simulink model "project_1"  (R2015b)
settings: Solver=ode15s  StartTime=0  StopTime=2000  FixedStep=1e-3  RelTol=1e-4
undefined symbols (not defined in the file): Kd_surge, Kd_sway, Kd_yaw, Ki_surge, Ki_sway, Ki_yaw, Kp_surge, Kp_sway, Kp_yaw, Par, Sim
libraries: marine_gnc x2
settings Model: Creator=torstebo  LastModifiedBy=ShivJeet
settings SolverCC: MaxConsecutiveMinStep=3  SolverJacobianMethodControl=FullPerturbation  ZeroCrossControl=DisableAll  ZeroCrossAlgorithm=Adaptive
settings DataIOCC: Decimation=10  InitialState=xFinal  LimitDataPoints=off  SaveFormat=StructureWithTime  SaveOutput=off  InspectSignalLogs=on  VisualizeSimOutput=off  SaveTime=off
settings OptimizationCC: AccelVerboseBuild=on
settings DebuggingCC: AlgebraicLoopMsg=error  UnderspecifiedInitializationDetection=Classic  MergeDetectMultiDrivingBlocksExec=none  SolverPrmCheckMsg=warning  StateNameClashWarn=warning
settings HardwareCC: ProdBitPerPointer=32  ProdLargestAtomicFloat=None  ProdIntDivRoundTo=Undefined  ProdEndianess=Unspecified  ProdWordSize=32  ProdHWDeviceType=32-bit Generic
settings GRTTargetCC: GeneratePreprocessorConditionals=Disable all
settings ConfigComp: CovModelRefEnable=Off  CovSFcnEnable=off

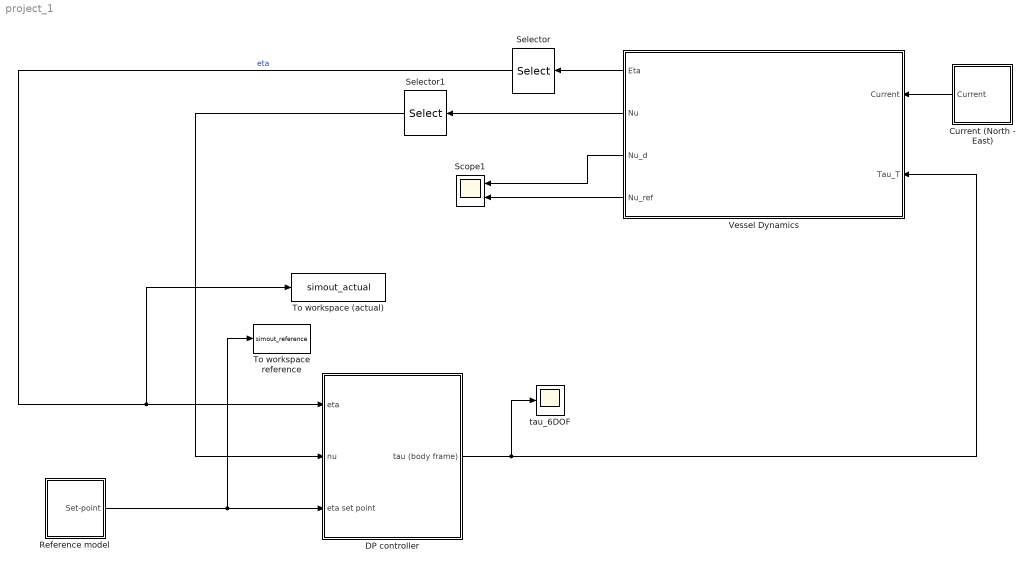
== system project_1 ==
  Current (North - East) : Subsystem
  DP controller : Subsystem
  Reference model : Subsystem
  Scope1 : Scope  NumInputPorts=2
  Selector : Selector  InputPortWidth=6  IndexOptions=Index vector (dialog)  Indices=[1 2 6]  OutputSizes=1
  Selector1 : Selector  InputPortWidth=6  IndexOptions=Index vector (dialog)  Indices=[1 2 6]  OutputSizes=1
  To workspace (actual) : ToWorkspace  VariableName=simout_actual  SaveFormat=Timeseries  SampleTime=-1
  To workspace reference : ToWorkspace  VariableName=simout_reference  SaveFormat=Timeseries  SampleTime=-1
  Vessel Dynamics : Subsystem
      mask Display:
      | image(imread('Files/supply.jpg'))
      | color('black'); port_label('output', 1, 'eta')
      | color('black'); port_label('output', 2, 'nu')
      | color('black'); port_label('output', 3, 'nu_d')
      | color('black'); port_label('output', 4, 'nu_ref')
      | color('black'); port_label('input', 1, 'nu_c')
      | color('black'); port_label('input', 2, 'tau')
  tau_6DOF : Scope
  wires:
  Vessel Dynamics/1(Eta) -> Selector/1
  Vessel Dynamics/2(Nu) -> Selector1/1
  Current (North - East)/1(Current) -> Vessel Dynamics/1(Current)
  DP controller/1(tau (body frame)) -> tau_6DOF/1, Vessel Dynamics/2(Tau_T)
  Reference model/1(Set-point) -> To workspace reference/1, DP controller/3(eta set point)
  Selector1/1 -> DP controller/2(nu)
  Vessel Dynamics/3(Nu_d) -> Scope1/1
  Vessel Dynamics/4(Nu_ref) -> Scope1/2
  Selector/1 -> To workspace (actual)/1, DP controller/1(eta)  "eta"

== system project_1/Current (North - East) ==
  Constant : Constant  Value=[0 0]
  Current : Outport
  wires:
  Constant/1 -> Current/1

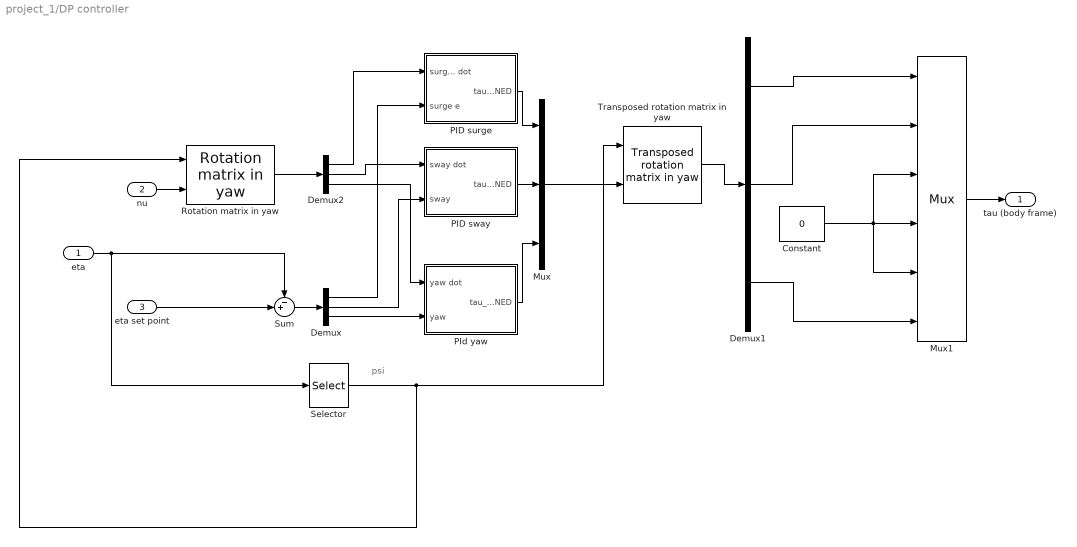
== system project_1/DP controller ==
  note: psi
  eta : Inport
  nu : Inport  Port=2
  eta set point : Inport  Port=3
  Constant : Constant  Value=0
  Demux : Demux  Outputs=3
  Demux1 : Demux  Outputs=3
  Demux2 : Demux  Outputs=3
  Mux : Mux  Inputs=3
  Mux1 : Mux  Inputs=6
  PID surge : Subsystem
  PID sway : Subsystem
  "PId yaw " : Subsystem
  "Rotation matrix in yaw " : marine_gnc/Models/ Kinematics/Rotation matrix in yaw 
  Selector : Selector  InputPortWidth=3  IndexOptions=Index vector (dialog)  Indices=3  OutputSizes=1
  Sum : Sum  Inputs=-+|
  Transposed rotation matrix in yaw : marine_gnc/Models/ Kinematics/Transposed rotation  matrix in yaw
  tau (body frame) : Outport
  wires:
  Sum/1 -> Demux/1
  eta/1 -> Sum/1, Selector/1
  eta set point/1 -> Sum/2
  Demux2/1 -> PID surge/1(surge dot)
  Demux/1 -> PID surge/2(surge e)
  Demux2/2 -> PID sway/1(sway dot)
  Demux2/3 -> "PId yaw "/1(yaw dot)
  Demux/2 -> PID sway/2(sway)
  Demux/3 -> "PId yaw "/2(yaw)
  "PId yaw "/1(tau_yaw_NED) -> Mux/3
  PID surge/1(tau_surge_NED) -> Mux/1
  PID sway/1(tau_sway_NED) -> Mux/2
  nu/1 -> "Rotation matrix in yaw "/2
  Selector/1 -> Transposed rotation matrix in yaw/1, "Rotation matrix in yaw "/1
  "Rotation matrix in yaw "/1 -> Demux2/1
  Constant/1 -> Mux1/3, Mux1/4, Mux1/5
  Mux1/1 -> tau (body frame)/1
  Transposed rotation matrix in yaw/1 -> Demux1/1
  Demux1/1 -> Mux1/1
  Demux1/2 -> Mux1/2
  Demux1/3 -> Mux1/6
  Mux/1 -> Transposed rotation matrix in yaw/2

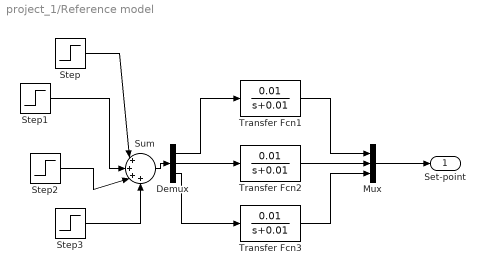
== system project_1/Reference model ==
  Demux : Demux  Outputs=3
  Mux : Mux  Inputs=3
  Step : Step  Time=50  Before=[0 0 0]  After=[10 0 0]  SampleTime=0
  Step1 : Step  Time=200  Before=[0 0 0]  After=[0 15 pi/2]  SampleTime=0
  Step2 : Step  Time=600  Before=[0 0 0]  After=[-10 0 pi/2]  SampleTime=0
  Step3 : Step  Time=1100  Before=[0 0 0]  After=[0 -15 pi/2]  SampleTime=0
  Sum : Sum  Inputs=|++++
  Transfer Fcn1 : TransferFcn  Numerator=[0.01]  Denominator=[1 0.01]
  Transfer Fcn2 : TransferFcn  Numerator=[0.01]  Denominator=[1 0.01]
  Transfer Fcn3 : TransferFcn  Numerator=[0.01]  Denominator=[1 0.01]
  Set-point : Outport
  wires:
  Mux/1 -> Set-point/1
  Transfer Fcn1/1 -> Mux/1
  Transfer Fcn2/1 -> Mux/2
  Transfer Fcn3/1 -> Mux/3
  Demux/1 -> Transfer Fcn1/1
  Demux/2 -> Transfer Fcn2/1
  Demux/3 -> Transfer Fcn3/1
  Sum/1 -> Demux/1
  Step3/1 -> Sum/4
  Step2/1 -> Sum/3
  Step1/1 -> Sum/2
  Step/1 -> Sum/1

== system project_1/Vessel Dynamics ==
  note: VESSEL MODULE
      | Consists of a WF and a LF module, which may be enabled or disabled in the Parameters file.
      | The LF and WFmotion components are written to the workspace for processing, and added for
      | use in the simulator.
  Current : Inport
  Tau_T : Inport  Port=2
  Vessel LF 6DOF : Subsystem
  Eta : Outport
  Nu : Outport  Port=2
  Nu_d : Outport  Port=3
  Nu_ref : Outport  Port=4
  wires:
  Current/1 -> Vessel LF 6DOF/2(Current_NED)
  Tau_T/1 -> Vessel LF 6DOF/1(External forces)  "Tau_T"
  Vessel LF 6DOF/1(Eta) -> Eta/1  "Eta_LF"
  Vessel LF 6DOF/2(Nu) -> Nu/1  "Nu_LF"
  Vessel LF 6DOF/3(Nu_d) -> Nu_d/1
  Vessel LF 6DOF/4(Nu_r) -> Nu_ref/1

== system project_1/DP controller/PID surge ==
  surge dot : Inport
  surge e : Inport  Port=2
  Gain1 : Gain  Gain=Kp_surge
  Gain2 : Gain  Gain=Ki_surge
  Integrator : Integrator
  Kd : Gain  Gain=Kd_surge
  Sum : Sum  Inputs=|-++
  tau_surge_NED : Outport
  wires:
  surge dot/1 -> Kd/1
  surge e/1 -> Gain1/1, Integrator/1
  Integrator/1 -> Gain2/1
  Kd/1 -> Sum/1
  Gain1/1 -> Sum/2
  Gain2/1 -> Sum/3
  Sum/1 -> tau_surge_NED/1

== system project_1/DP controller/PID sway ==
  sway dot : Inport
  sway : Inport  Port=2
  Integrator : Integrator
  Kd : Gain  Gain=Kd_sway
  Ki : Gain  Gain=Ki_sway
  Kp : Gain  Gain=Kp_sway
  Sum : Sum  Inputs=|-++
  tau_sway_NED : Outport
  wires:
  sway dot/1 -> Kd/1
  sway/1 -> Kp/1, Integrator/1
  Integrator/1 -> Ki/1
  Kd/1 -> Sum/1
  Kp/1 -> Sum/2
  Ki/1 -> Sum/3
  Sum/1 -> tau_sway_NED/1

== system project_1/DP controller/PId yaw  ==
  yaw dot : Inport
  yaw : Inport  Port=2
  Gain : Gain  Gain=Kd_yaw
  Gain1 : Gain  Gain=Kp_yaw
  Gain2 : Gain  Gain=Ki_yaw
  Integrator : Integrator
  Sum : Sum  Inputs=|-++
  tau_yaw_NED : Outport
  wires:
  yaw dot/1 -> Gain/1
  yaw/1 -> Gain1/1, Integrator/1
  Integrator/1 -> Gain2/1
  Gain/1 -> Sum/1
  Gain1/1 -> Sum/2
  Gain2/1 -> Sum/3
  Sum/1 -> tau_yaw_NED/1

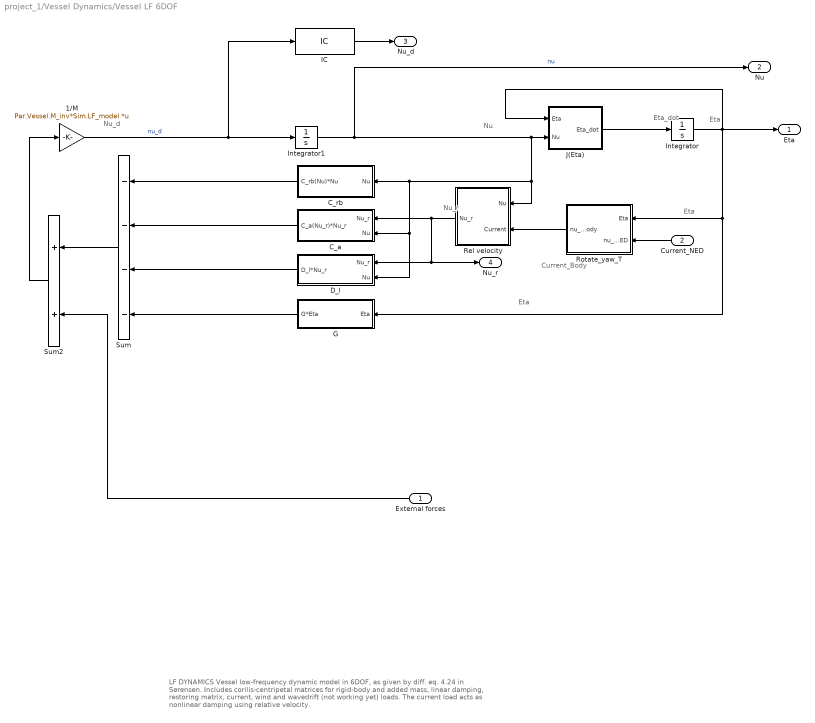
== system project_1/Vessel Dynamics/Vessel LF 6DOF ==
  note: Nu_d
  note: Nu
  note: Eta
  note: Current_Body
  note: Eta
  note: Nu_r
  note: Eta
  note: LF DYNAMICS
      | Vessel low-frequency dynamic model in 6DOF, as given by diff. eq. 4.24 in Sørensen.
      | Includes corilis-centripetal matrices for rigid-body and added mass, linear damping,
      | restoring matrix, current, wind and wavedrift (not working yet) loads. The current load
      | acts as nonlinear damping using relative velocity.
  note: Eta_dot
  External forces : Inport
  Current_NED : Inport  Port=2
  1/M : Gain  Gain=Par.Vessel.M_inv*Sim.LF_model  Multiplication=Matrix(K*u) (u vector)  SaturateOnIntegerOverflow=on  OutDataTypeStr=Inherit: Same as input  ParamDataTypeStr=Inherit: Same as input
  C_a : Subsystem
  C_rb : Subsystem
  D_l : Subsystem
      settings: MinAlgLoopOccurrences=on
  G : Subsystem
  IC : InitialCondition  Value=Sim.Nu_d_init
  Integrator : Integrator  InitialCondition=Sim.Eta_init
  Integrator1 : Integrator  InitialCondition=Sim.Nu_init
  J(Eta) : Subsystem
  Rel velocity : Subsystem
  Rotate_yaw_T : Subsystem
  Sum : Sum  Inputs=----  SaturateOnIntegerOverflow=on
  Sum2 : Sum  SaturateOnIntegerOverflow=on
  Eta : Outport
  Nu : Outport  Port=2
  Nu_d : Outport  Port=3
  Nu_r : Outport  Port=4
  wires:
  1/M/1 -> IC/1, Integrator1/1  "nu_d"
  J(Eta)/1(Eta_dot) -> Integrator/1
  Integrator/1 -> J(Eta)/1(Eta), Eta/1, Rotate_yaw_T/1(Eta), G/1(Eta)
  Integrator1/1 -> Nu/1, J(Eta)/2(Nu), Rel velocity/1(Nu), C_a/2(Nu), D_l/2(Nu), C_rb/1(Nu)  "nu"
  Current_NED/1 -> Rotate_yaw_T/2(nu_2D_NED)
  Rotate_yaw_T/1(nu_2D_body) -> Rel velocity/2(Current)
  Rel velocity/1(Nu_r) -> D_l/1(Nu_r), Nu_r/1, C_a/1(Nu_r)
  Sum/1 -> Sum2/1
  External forces/1 -> Sum2/2
  Sum2/1 -> 1/M/1
  C_rb/1(C_rb(Nu)*Nu) -> Sum/1
  C_a/1(C_a(Nu_r)*Nu_r) -> Sum/2
  D_l/1(D_l*Nu_r) -> Sum/3
  G/1(G*Eta) -> Sum/4
  IC/1 -> Nu_d/1

== system project_1/Vessel Dynamics/Vessel LF 6DOF/C_a ==
  note: C_a
      | Coriolis-centripetal added mass force calculation using the S-function m2c_S.
      | This effect can be included/excluded from the Parameters file.
      | A choice of using absolute or relative vessel velocity is also given.
      | OS2002
  Nu_r : Inport
  Nu : Inport  Port=2
  C_a calculation : Subsystem  TreatAsAtomicUnit=on
  Enable Coriolis added mass force : Constant  Value=Sim.C_a
  Sim.Nu_r_C_a : Constant  Value=Sim.Nu_r_C_a
  Switch : Switch  Criteria=u2 > Threshold  SaturateOnIntegerOverflow=on
  C_a(Nu_r)*Nu_r : Outport
  wires:
  C_a calculation/1(F) -> C_a(Nu_r)*Nu_r/1
  Nu_r/1 -> Switch/1
  Nu/1 -> Switch/3
  Sim.Nu_r_C_a/1 -> Switch/2
  Switch/1 -> C_a calculation/1(Nu_r)
  Enable Coriolis added mass force/1 -> C_a calculation/Enable

== system project_1/Vessel Dynamics/Vessel LF 6DOF/C_rb ==
  note: C_rb
      | Coriolis-centripetal rigid-body force calculation using the S-function m2c_S.
      | This effect can be included/excluded from the Parameters file.
      | OS2002
  Nu : Inport
  C_rb Calculation : Subsystem  TreatAsAtomicUnit=on
  Enable Coriolis added mass force : Constant  Value=Sim.C_rb
  C_rb(Nu)*Nu : Outport
  wires:
  Nu/1 -> C_rb Calculation/1(Nu_r)
  Enable Coriolis added mass force/1 -> C_rb Calculation/Enable
  C_rb Calculation/1(F) -> C_rb(Nu)*Nu/1

== system project_1/Vessel Dynamics/Vessel LF 6DOF/D_l ==
  note: D_l
      | Linear damping, matrix formulation.
      | This effect can be included/excluded from the Parameters file.
      | A choice of using absolute or relative vessel velocity is also given.
      | OS2002
  Nu_r : Inport
  Nu : Inport  Port=2
  D_l : Gain  Gain=Par.Vessel.DL  Multiplication=Matrix(K*u)  SaturateOnIntegerOverflow=on  OutDataTypeStr=Inherit: Same as input  ParamDataTypeStr=Inherit: Same as input
  Include D_l : Gain  Gain=Sim.D_l  SaturateOnIntegerOverflow=on  OutDataTypeStr=Inherit: Same as input  ParamDataTypeStr=Inherit: Same as input
  Sim.Nu_r_D_l : Constant  Value=Sim.Nu_r_D_l
  Switch : Switch  Criteria=u2 > Threshold  SaturateOnIntegerOverflow=on
  D_l*Nu_r : Outport
  wires:
  D_l/1 -> Include D_l/1
  Include D_l/1 -> D_l*Nu_r/1
  Switch/1 -> D_l/1
  Nu_r/1 -> Switch/1
  Nu/1 -> Switch/3
  Sim.Nu_r_D_l/1 -> Switch/2

== system project_1/Vessel Dynamics/Vessel LF 6DOF/G ==
  note: G
      | Standard restoring matrix. This effect can
      | be included/excluded from the Parameters file.
      | OS2002
  Eta : Inport
  G : Gain  Gain=Par.Vessel.G  Multiplication=Matrix(K*u)  SaturateOnIntegerOverflow=on  OutDataTypeStr=Inherit: Same as input  ParamDataTypeStr=Inherit: Same as input
  Include G : Gain  Gain=Sim.G  SaturateOnIntegerOverflow=on  OutDataTypeStr=Inherit: Same as input  ParamDataTypeStr=Inherit: Same as input
  G*Eta : Outport
  wires:
  Eta/1 -> G/1
  G/1 -> Include G/1
  Include G/1 -> G*Eta/1

== system project_1/Vessel Dynamics/Vessel LF 6DOF/J(Eta) ==
  note: Theta
  note: v
  note: omega
  note: J(Eta)
      | Standard 6DOF rotation matrix, as defined by Fossen. Using the two
      | rotation matrices Rnb and Tnb from the gnc Simulink toolbox.
      | OS2002
  Eta : Inport
  Nu : Inport  Port=2
  Mux : Mux  Inputs=2
  Product : Product  Inputs=**  Multiplication=Matrix(*)  SaturateOnIntegerOverflow=on  OutDataTypeStr=Inherit: Same as first input
  Product1 : Product  Inputs=**  Multiplication=Matrix(*)  SaturateOnIntegerOverflow=on  OutDataTypeStr=Inherit: Same as first input
  Rnb_gnc : Subsystem
  Selector : Selector  InputPortWidth=6  IndexOptions=Index vector (dialog)  Indices=[4 5 6]  OutputSizes=1
  Selector1 : Selector  InputPortWidth=6  IndexOptions=Index vector (dialog)  Indices=[1 2 3]  OutputSizes=1
  Selector2 : Selector  InputPortWidth=6  IndexOptions=Index vector (dialog)  Indices=[4 5 6]  OutputSizes=1
  Tnb_gnc : Subsystem
  Eta_dot : Outport
  wires:
  Selector/1 -> Tnb_gnc/1(theta), Rnb_gnc/1(theta)
  Eta/1 -> Selector/1
  Rnb_gnc/1(Rzyx) -> Product/1
  Nu/1 -> Selector1/1, Selector2/1
  Selector1/1 -> Product/2
  Selector2/1 -> Product1/2
  Tnb_gnc/1(T) -> Product1/1
  Product/1 -> Mux/1
  Mux/1 -> Eta_dot/1
  Product1/1 -> Mux/2

== system project_1/Vessel Dynamics/Vessel LF 6DOF/Rel velocity ==
  note: REL VELOCITY
      | Calculate relative vessel velociy
      | including current.
      | OS2002
  Nu : Inport
  Current : Inport  Port=2
  Mux : Mux  Inputs=2
  Sum : Sum  Inputs=+-  SaturateOnIntegerOverflow=on
  Zeros : Constant  Value=[0 0 0 0]
  Nu_r : Outport
  wires:
  Current/1 -> Mux/1
  Nu/1 -> Sum/1
  Sum/1 -> Nu_r/1
  Mux/1 -> Sum/2
  Zeros/1 -> Mux/2

== system project_1/Vessel Dynamics/Vessel LF 6DOF/Rotate_yaw_T ==
  note: ROTATE_YAW_T
      | The transposed rotation matrix in yaw, as defined
      | by Fossen. Rotates a velocity or coordinate a positive
      | yaw angle. Corresponds to matlab function  rotate_yaw_T
      | by OS. Uses the gcn Simulink function GNC: "Transposed
      | rotation matrix yaw"
      | OS2002
  Eta : Inport
  nu_2D_NED : Inport  Port=2
  "GNC: \"Transposed rotation matrix yaw\"" : Subsystem
  Mux : Mux  Inputs=2
  Selector : Selector  InputPortWidth=3  IndexOptions=Index vector (dialog)  Indices=[1 2]  OutputSizes=1
  Selector1 : Selector  InputPortWidth=6  IndexOptions=Index vector (dialog)  Indices=6  OutputSizes=1
  psi : Constant  Value=0
  nu_2D_body : Outport
  wires:
  Selector1/1 -> "GNC: \"Transposed rotation matrix yaw\""/1(psi)
  nu_2D_NED/1 -> Mux/1
  psi/1 -> Mux/2
  "GNC: \"Transposed rotation matrix yaw\""/1(R*nu) -> Selector/1
  Selector/1 -> nu_2D_body/1
  Eta/1 -> Selector1/1
  Mux/1 -> "GNC: \"Transposed rotation matrix yaw\""/2(nu)

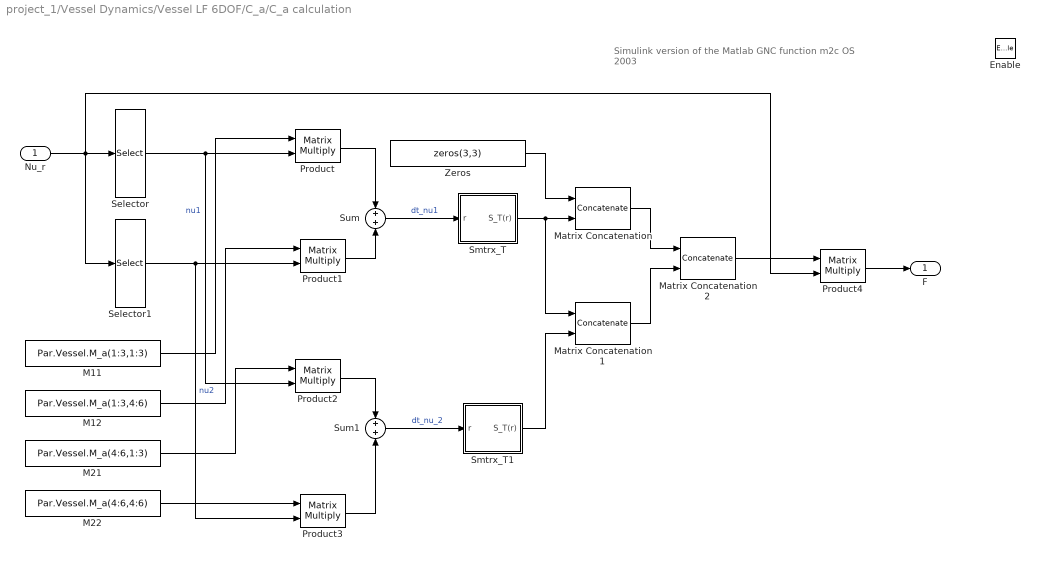
== system project_1/Vessel Dynamics/Vessel LF 6DOF/C_a/C_a calculation ==
  note: Simulink version of the Matlab GNC function m2c
      | OS 2003
  Nu_r : Inport
  Enable : EnablePort
  M11 : Constant  Value=Par.Vessel.M_a(1:3,1:3)
  M12 : Constant  Value=Par.Vessel.M_a(1:3,4:6)
  M21 : Constant  Value=Par.Vessel.M_a(4:6,1:3)
  M22 : Constant  Value=Par.Vessel.M_a(4:6,4:6)
  Matrix Concatenation : Concatenate  Mode=Multidimensional array  ConcatenateDimension=2
  Matrix Concatenation1 : Concatenate  Mode=Multidimensional array  ConcatenateDimension=2
  Matrix Concatenation2 : Concatenate  Mode=Multidimensional array
  Product{,1..4} (5 alike) : Product  Multiplication=Matrix(*)  SaturateOnIntegerOverflow=on  OutDataTypeStr=Inherit: Same as first input
  Selector : Selector  InputPortWidth=6  IndexOptions=Index vector (dialog)  Indices=[1:3]  OutputSizes=1
  Selector1 : Selector  InputPortWidth=6  IndexOptions=Index vector (dialog)  Indices=[4:6]  OutputSizes=1
  Smtrx_T : Subsystem
  Smtrx_T1 : Subsystem
  Sum : Sum  Inputs=+|+  SaturateOnIntegerOverflow=on
  Sum1 : Sum  Inputs=+|+  SaturateOnIntegerOverflow=on
  Zeros : Constant  Value=zeros(3,3)
  F : Outport
  wires:
  Nu_r/1 -> Selector/1, Selector1/1, Product4/2
  Product/1 -> Sum/1
  Product1/1 -> Sum/2
  Product2/1 -> Sum1/1
  Product3/1 -> Sum1/2
  Sum/1 -> Smtrx_T/1(r)  "dt_nu1"
  Sum1/1 -> Smtrx_T1/1(r)  "dt_nu_2"
  Zeros/1 -> Matrix Concatenation/1
  Smtrx_T/1(S_T(r)) -> Matrix Concatenation/2, Matrix Concatenation1/1
  Smtrx_T1/1(S_T(r)) -> Matrix Concatenation1/2
  Matrix Concatenation/1 -> Matrix Concatenation2/1
  Matrix Concatenation1/1 -> Matrix Concatenation2/2
  Product4/1 -> F/1
  Selector/1 -> Product/2, Product2/2  "nu1"
  Selector1/1 -> Product1/2, Product3/2  "nu2"
  M11/1 -> Product/1
  M12/1 -> Product1/1
  M22/1 -> Product3/1
  M21/1 -> Product2/1
  Matrix Concatenation2/1 -> Product4/1

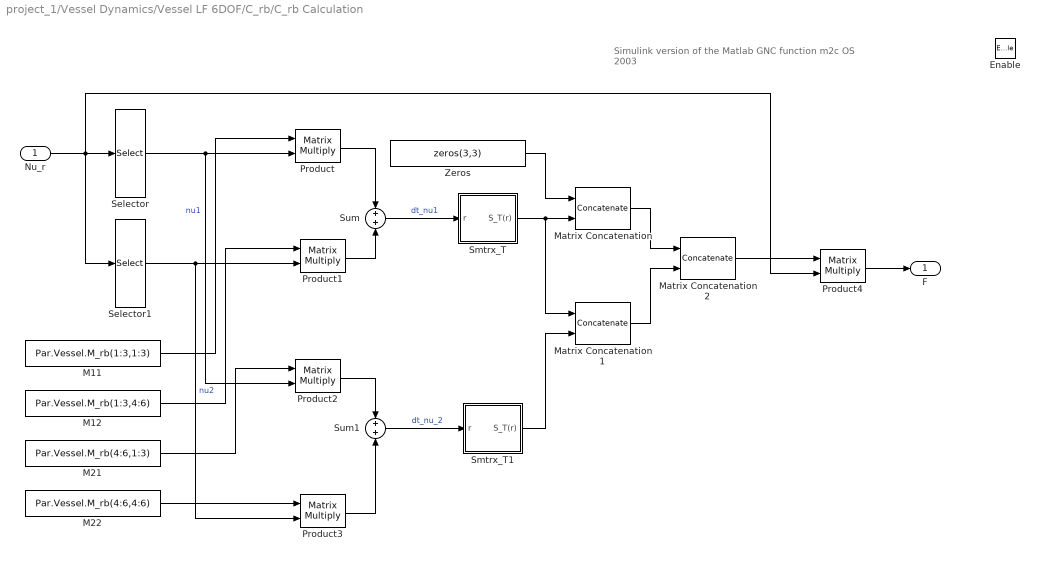
== system project_1/Vessel Dynamics/Vessel LF 6DOF/C_rb/C_rb Calculation ==
  note: Simulink version of the Matlab GNC function m2c
      | OS 2003
  Nu_r : Inport
  Enable : EnablePort
  M11 : Constant  Value=Par.Vessel.M_rb(1:3,1:3)
  M12 : Constant  Value=Par.Vessel.M_rb(1:3,4:6)
  M21 : Constant  Value=Par.Vessel.M_rb(4:6,1:3)
  M22 : Constant  Value=Par.Vessel.M_rb(4:6,4:6)
  Matrix Concatenation : Concatenate  Mode=Multidimensional array  ConcatenateDimension=2
  Matrix Concatenation1 : Concatenate  Mode=Multidimensional array  ConcatenateDimension=2
  Matrix Concatenation2 : Concatenate  Mode=Multidimensional array
  Product{,1..4} (5 alike) : Product  Multiplication=Matrix(*)  SaturateOnIntegerOverflow=on  OutDataTypeStr=Inherit: Same as first input
  Selector : Selector  InputPortWidth=6  IndexOptions=Index vector (dialog)  Indices=[1:3]  OutputSizes=1
  Selector1 : Selector  InputPortWidth=6  IndexOptions=Index vector (dialog)  Indices=[4:6]  OutputSizes=1
  Smtrx_T : Subsystem
  Smtrx_T1 : Subsystem
  Sum : Sum  Inputs=+|+  SaturateOnIntegerOverflow=on
  Sum1 : Sum  Inputs=+|+  SaturateOnIntegerOverflow=on
  Zeros : Constant  Value=zeros(3,3)
  F : Outport
  wires:
  Nu_r/1 -> Selector/1, Selector1/1, Product4/2
  Product/1 -> Sum/1
  Product1/1 -> Sum/2
  Product2/1 -> Sum1/1
  Product3/1 -> Sum1/2
  Sum/1 -> Smtrx_T/1(r)  "dt_nu1"
  Sum1/1 -> Smtrx_T1/1(r)  "dt_nu_2"
  Zeros/1 -> Matrix Concatenation/1
  Smtrx_T/1(S_T(r)) -> Matrix Concatenation/2, Matrix Concatenation1/1
  Smtrx_T1/1(S_T(r)) -> Matrix Concatenation1/2
  Matrix Concatenation/1 -> Matrix Concatenation2/1
  Matrix Concatenation1/1 -> Matrix Concatenation2/2
  Product4/1 -> F/1
  Selector/1 -> Product/2, Product2/2  "nu1"
  Selector1/1 -> Product1/2, Product3/2  "nu2"
  M11/1 -> Product/1
  M12/1 -> Product1/1
  M22/1 -> Product3/1
  M21/1 -> Product2/1
  Matrix Concatenation2/1 -> Product4/1

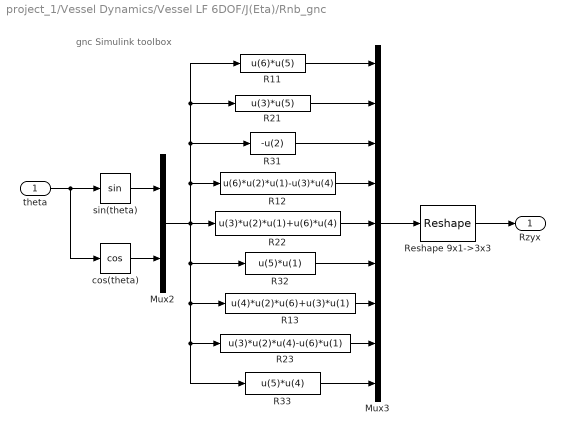
== system project_1/Vessel Dynamics/Vessel LF 6DOF/J(Eta)/Rnb_gnc ==
  note: gnc Simulink toolbox
  theta : Inport
  Mux2 : Mux  Inputs=2
  Mux3 : Mux  Inputs=9
  R11 : Fcn  Expr=u(6)*u(5)
  R12 : Fcn  Expr=u(6)*u(2)*u(1)-u(3)*u(4)
  R13 : Fcn  Expr=u(4)*u(2)*u(6)+u(3)*u(1)
  "R21 " : Fcn  Expr=u(3)*u(5)
  R22 : Fcn  Expr=u(3)*u(2)*u(1)+u(6)*u(4)
  R23 : Fcn  Expr=u(3)*u(2)*u(4)-u(6)*u(1)
  "R31 " : Fcn  Expr=-u(2)
  R32 : Fcn  Expr=u(5)*u(1)
  R33 : Fcn  Expr=u(5)*u(4)
  Reshape 9x1->3x3 : Reshape  OutputDimensionality=Customize  OutputDimensions=[3,3]
  cos(theta) : Trigonometry  Operator=cos
  sin(theta) : Trigonometry
  Rzyx : Outport  InitialOutput=0
  wires:
  R11/1 -> Mux3/1
  Mux3/1 -> Reshape 9x1->3x3/1
  Reshape 9x1->3x3/1 -> Rzyx/1
  sin(theta)/1 -> Mux2/1
  cos(theta)/1 -> Mux2/2
  theta/1 -> cos(theta)/1, sin(theta)/1
  Mux2/1 -> R32/1, R13/1, R33/1, R23/1, R22/1, "R31 "/1, R11/1, "R21 "/1, R12/1
  R23/1 -> Mux3/8
  R13/1 -> Mux3/7
  R22/1 -> Mux3/5
  R12/1 -> Mux3/4
  "R31 "/1 -> Mux3/3
  "R21 "/1 -> Mux3/2
  R32/1 -> Mux3/6
  R33/1 -> Mux3/9

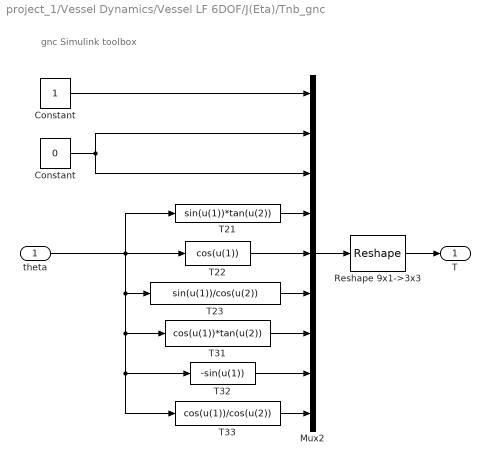
== system project_1/Vessel Dynamics/Vessel LF 6DOF/J(Eta)/Tnb_gnc ==
  note: gnc Simulink toolbox
  theta : Inport
  Constant : Constant
  "Constant " : Constant  Value=0
  Mux2 : Mux  Inputs=9
  Reshape 9x1->3x3 : Reshape  OutputDimensionality=Customize  OutputDimensions=[3,3]
  "T21 " : Fcn  Expr=sin(u(1))*tan(u(2))
  T22 : Fcn  Expr=cos(u(1))
  T23 : Fcn  Expr=sin(u(1))/cos(u(2))
  "T31 " : Fcn  Expr=cos(u(1))*tan(u(2))
  T32 : Fcn  Expr=-sin(u(1))
  T33 : Fcn  Expr=cos(u(1))/cos(u(2))
  T : Outport  InitialOutput=0
  wires:
  Constant/1 -> Mux2/1
  Mux2/1 -> Reshape 9x1->3x3/1
  Reshape 9x1->3x3/1 -> T/1
  theta/1 -> "T21 "/1, T22/1, "T31 "/1, T32/1, T33/1, T23/1
  T23/1 -> Mux2/6
  T22/1 -> Mux2/5
  T33/1 -> Mux2/9
  "Constant "/1 -> Mux2/2, Mux2/3
  "T21 "/1 -> Mux2/4
  "T31 "/1 -> Mux2/7
  T32/1 -> Mux2/8

== system project_1/Vessel Dynamics/Vessel LF 6DOF/Rotate_yaw_T/GNC: "Transposed rotation matrix yaw" ==
  note: GNC: "Transposed
      | rotation matrix yaw"
  psi : Inport
  nu : Inport  Port=2  PortDimensions=3
  Fcn : Fcn  Expr=cos(u(1))*u(2)+sin(u(1))*u(3)
  Fcn1 : Fcn  Expr=-sin(u(1))*u(2)+cos(u(1))*u(3)
  Fcn2 : Fcn  Expr=u(4)
  Mux2 : Mux  Inputs=2
  Mux3 : Mux  Inputs=3
  R*nu : Outport
  wires:
  Mux2/1 -> Fcn1/1, Fcn/1, Fcn2/1
  Fcn/1 -> Mux3/1  "x_dot"
  Fcn1/1 -> Mux3/2  "y_dot"
  Fcn2/1 -> Mux3/3  "psi_dot"
  Mux3/1 -> R*nu/1  "eta_dot"
  psi/1 -> Mux2/1
  nu/1 -> Mux2/2

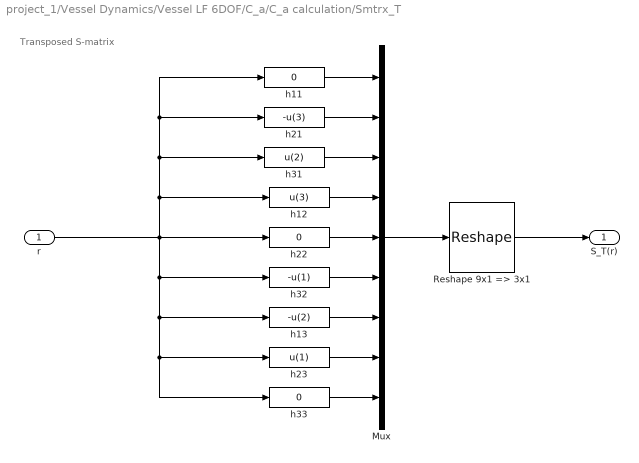
== system project_1/Vessel Dynamics/Vessel LF 6DOF/C_a/C_a calculation/Smtrx_T ==
  note: Transposed S-matrix
  r : Inport
  Mux : Mux  Inputs=9
  Reshape 9x1 => 3x1 : Reshape  OutputDimensionality=Customize  OutputDimensions=[3,3]
  h11 : Fcn  Expr=0
  h12 : Fcn  Expr=u(3)
  h13 : Fcn  Expr=-u(2)
  h21 : Fcn  Expr=-u(3)
  h22 : Fcn  Expr=0
  h23 : Fcn  Expr=u(1)
  h31 : Fcn  Expr=u(2)
  h32 : Fcn  Expr=-u(1)
  h33 : Fcn  Expr=0
  S_T(r) : Outport
  wires:
  r/1 -> h33/1, h23/1, h13/1, h32/1, h22/1, h12/1, h21/1, h11/1, h31/1
  h33/1 -> Mux/9
  h23/1 -> Mux/8
  h13/1 -> Mux/7
  h32/1 -> Mux/6
  h22/1 -> Mux/5
  h12/1 -> Mux/4
  h31/1 -> Mux/3
  h21/1 -> Mux/2
  h11/1 -> Mux/1
  Mux/1 -> Reshape 9x1 => 3x1/1
  Reshape 9x1 => 3x1/1 -> S_T(r)/1

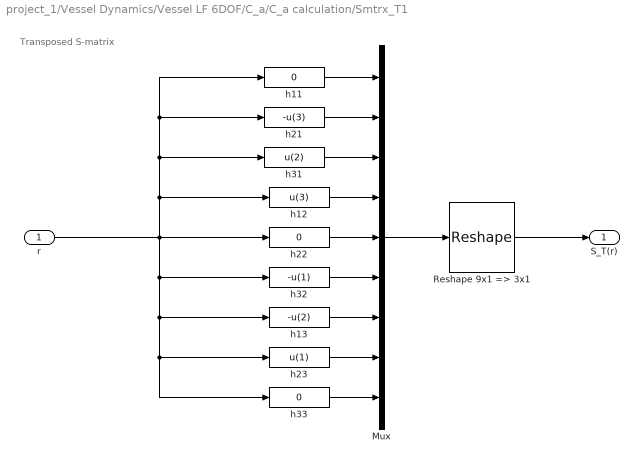
== system project_1/Vessel Dynamics/Vessel LF 6DOF/C_a/C_a calculation/Smtrx_T1 ==
  note: Transposed S-matrix
  r : Inport
  Mux : Mux  Inputs=9
  Reshape 9x1 => 3x1 : Reshape  OutputDimensionality=Customize  OutputDimensions=[3,3]
  h11 : Fcn  Expr=0
  h12 : Fcn  Expr=u(3)
  h13 : Fcn  Expr=-u(2)
  h21 : Fcn  Expr=-u(3)
  h22 : Fcn  Expr=0
  h23 : Fcn  Expr=u(1)
  h31 : Fcn  Expr=u(2)
  h32 : Fcn  Expr=-u(1)
  h33 : Fcn  Expr=0
  S_T(r) : Outport
  wires:
  Reshape 9x1 => 3x1/1 -> S_T(r)/1
  Mux/1 -> Reshape 9x1 => 3x1/1
  h11/1 -> Mux/1
  h21/1 -> Mux/2
  h31/1 -> Mux/3
  h12/1 -> Mux/4
  h22/1 -> Mux/5
  h32/1 -> Mux/6
  h13/1 -> Mux/7
  h23/1 -> Mux/8
  h33/1 -> Mux/9
  r/1 -> h31/1, h11/1, h21/1, h12/1, h22/1, h32/1, h13/1, h23/1, h33/1

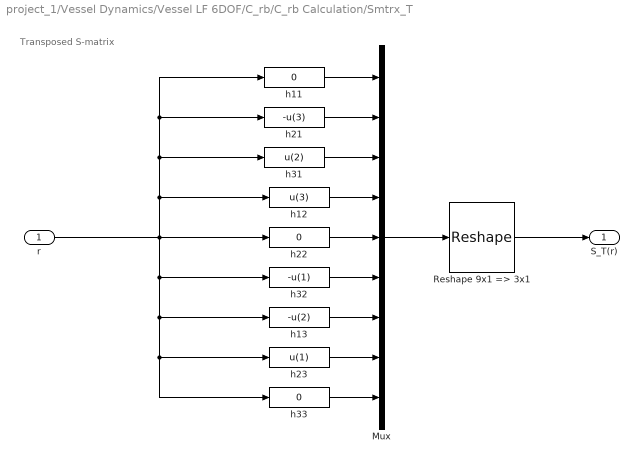
== system project_1/Vessel Dynamics/Vessel LF 6DOF/C_rb/C_rb Calculation/Smtrx_T ==
  note: Transposed S-matrix
  r : Inport
  Mux : Mux  Inputs=9
  Reshape 9x1 => 3x1 : Reshape  OutputDimensionality=Customize  OutputDimensions=[3,3]
  h11 : Fcn  Expr=0
  h12 : Fcn  Expr=u(3)
  h13 : Fcn  Expr=-u(2)
  h21 : Fcn  Expr=-u(3)
  h22 : Fcn  Expr=0
  h23 : Fcn  Expr=u(1)
  h31 : Fcn  Expr=u(2)
  h32 : Fcn  Expr=-u(1)
  h33 : Fcn  Expr=0
  S_T(r) : Outport
  wires:
  r/1 -> h22/1, h12/1, h21/1, h11/1, h31/1, h33/1, h23/1, h13/1, h32/1
  h33/1 -> Mux/9
  h23/1 -> Mux/8
  h13/1 -> Mux/7
  h32/1 -> Mux/6
  h22/1 -> Mux/5
  h12/1 -> Mux/4
  h31/1 -> Mux/3
  h21/1 -> Mux/2
  h11/1 -> Mux/1
  Mux/1 -> Reshape 9x1 => 3x1/1
  Reshape 9x1 => 3x1/1 -> S_T(r)/1

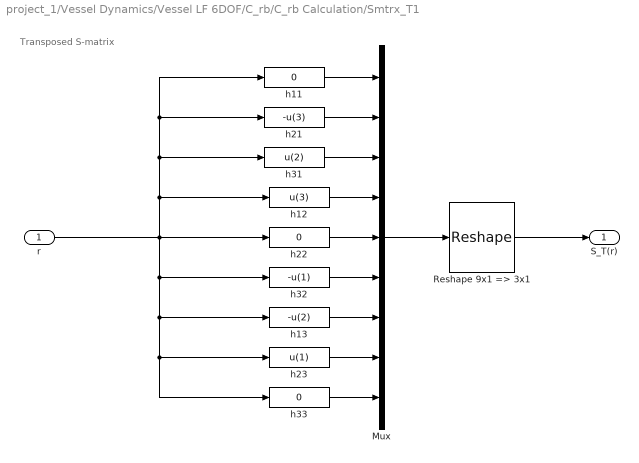
== system project_1/Vessel Dynamics/Vessel LF 6DOF/C_rb/C_rb Calculation/Smtrx_T1 ==
  note: Transposed S-matrix
  r : Inport
  Mux : Mux  Inputs=9
  Reshape 9x1 => 3x1 : Reshape  OutputDimensionality=Customize  OutputDimensions=[3,3]
  h11 : Fcn  Expr=0
  h12 : Fcn  Expr=u(3)
  h13 : Fcn  Expr=-u(2)
  h21 : Fcn  Expr=-u(3)
  h22 : Fcn  Expr=0
  h23 : Fcn  Expr=u(1)
  h31 : Fcn  Expr=u(2)
  h32 : Fcn  Expr=-u(1)
  h33 : Fcn  Expr=0
  S_T(r) : Outport
  wires:
  Reshape 9x1 => 3x1/1 -> S_T(r)/1
  Mux/1 -> Reshape 9x1 => 3x1/1
  h11/1 -> Mux/1
  h21/1 -> Mux/2
  h31/1 -> Mux/3
  h12/1 -> Mux/4
  h22/1 -> Mux/5
  h32/1 -> Mux/6
  h13/1 -> Mux/7
  h23/1 -> Mux/8
  h33/1 -> Mux/9
  r/1 -> h31/1, h11/1, h21/1, h12/1, h22/1, h32/1, h13/1, h23/1, h33/1
